simulink library "INT_CoEng_Mon"  (R2016b)
settings: Solver=VariableStepAuto  StartTime=0.0  StopTime=10.0  RelTol=1e-3
settings Model: Creator=Administrator  LastModifiedBy=Administrator

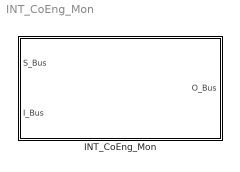
== system INT_CoEng_Mon ==
  INT_CoEng_Mon : Subsystem

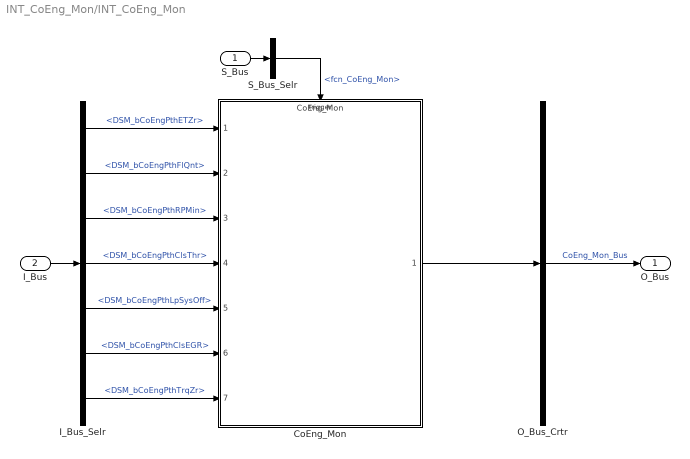
== system INT_CoEng_Mon/INT_CoEng_Mon ==
  S_Bus : Inport
  I_Bus : Inport  Port=2
  CoEng_Mon : ModelReference  ModelNameDialog=CoEng_Mon  SimulationMode=Normal  ModelReferenceVersion=1.2  TriggerPortName=function  TriggerPortTriggerType=function-call  TriggerPortStatesWhenEnabling=held
  I_Bus_Selr : BusSelector  OutputSignals=DSM_bCoEngPthETZr,DSM_bCoEngPthFlQnt,DSM_bCoEngPthRPMin,DSM_bCoEngPthClsThr,DSM_bCoEngPthLpSysOff,DSM_bCoEngPthClsEGR,DSM_bCoEngPthTrqZr
  O_Bus_Crtr : BusCreator  Inputs=1
  S_Bus_Selr : BusSelector  OutputSignals=fcn_CoEng_Mon
  O_Bus : Outport
  wires:
  S_Bus_Selr/1 -> CoEng_Mon/Trigger  "<fcn_CoEng_Mon>"
  S_Bus/1 -> S_Bus_Selr/1
  I_Bus/1 -> I_Bus_Selr/1
  I_Bus_Selr/1 -> CoEng_Mon/1  "<DSM_bCoEngPthETZr>"
  I_Bus_Selr/2 -> CoEng_Mon/2  "<DSM_bCoEngPthFlQnt>"
  I_Bus_Selr/3 -> CoEng_Mon/3  "<DSM_bCoEngPthRPMin>"
  I_Bus_Selr/4 -> CoEng_Mon/4  "<DSM_bCoEngPthClsThr>"
  I_Bus_Selr/5 -> CoEng_Mon/5  "<DSM_bCoEngPthLpSysOff>"
  I_Bus_Selr/6 -> CoEng_Mon/6  "<DSM_bCoEngPthClsEGR>"
  I_Bus_Selr/7 -> CoEng_Mon/7  "<DSM_bCoEngPthTrqZr>"
  O_Bus_Crtr/1 -> O_Bus/1  "CoEng_Mon_Bus"
  CoEng_Mon/1 -> O_Bus_Crtr/1
